simulink model "gm_interlock_deadtime_vnl"  (R2020b)
settings: Solver=FixedStepDiscrete  StartTime=0.0  StopTime=0.01  RelTol=1e-3
libraries: simulink x17, hdlmdlgenlib x12, hdlsllib x7, eePwmGeneratorTwoLevel x1, powerlib_meascontrol x1
(part 1 of 2)
settings Model: Creator=ts  LastModifiedBy=ts
settings DataIOCC: LimitDataPoints=on  SaveOutput=off  SaveTime=off
settings OptimizationCC: BlockReduction=off  ConditionallyExecuteInputs=off  DefaultParameterBehavior=Inlined  LifeSpan=inf
settings DebuggingCC: AlgebraicLoopMsg=error  InheritedTsInSrcMsg=none  SingleTaskRateTransMsg=error  AllowSymbolicDim=off  StrictBusMsg=ErrorOnBusTreatedAsVector  SFUnexpectedBacktrackingDiag=warning  SFNoUnconditionalDefaultTransitionDiag=warning  SFExecutionAtInitializationDiag=none  ArithmeticOperatorsInVariantConditions=warning
settings HardwareCC: ProdBitPerPointer=32  ProdBitPerSizeT=32  ProdBitPerPtrDiffT=32  ProdLargestAtomicFloat=None  ProdIntDivRoundTo=Undefined  ProdEndianess=Unspecified  ProdWordSize=32  ProdHWDeviceType=ASIC/FPGA->ASIC/FPGA  ProdEqTarget=off
settings SFSimCC: SimUseLocalCustomCode=off  CustomCodeUndefinedFunction=UseInterfaceOnly
settings RTWCC: RTWUseLocalCustomCode=off
settings CodeAppCC: StateflowObjectComments=on
settings GRTTargetCC: TargetLangStandard=C89/C90 (ANSI)
settings ConfigComp: CovScope=ReferencedModels  CovMetricSettings=dw  CovSaveCumulativeToWorkspaceVar=on  CovSaveSingleToWorkspaceVar=on  CovExternalEMLEnable=off  CovSFcnEnable=off

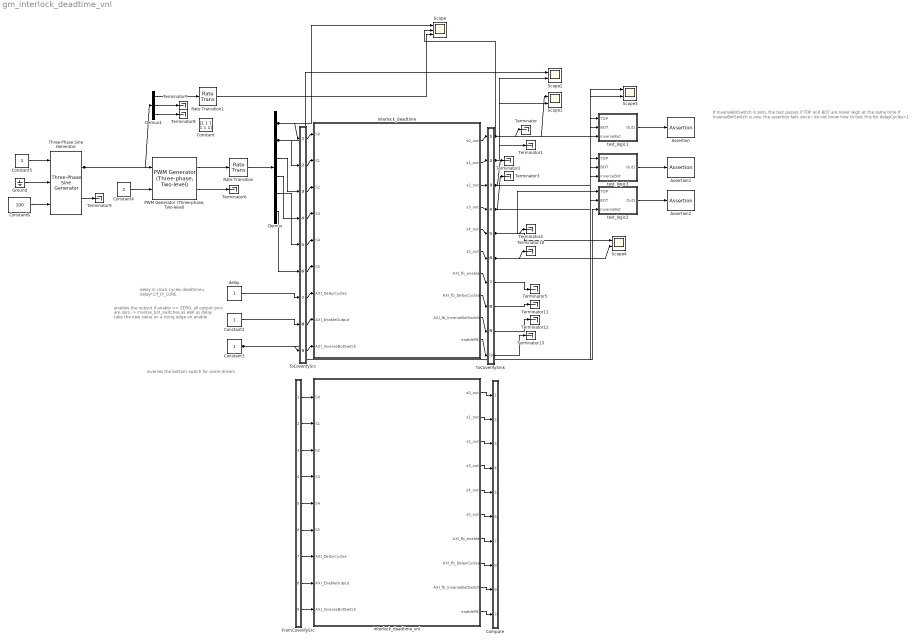
== system gm_interlock_deadtime_vnl ==
  note: If InverseBotSwitch is zero, the test passes if TOP and BOT are never High at the same time
      | If InverseBotSwitch is one, the assertion fails since I do not know how to test this for delayCycles>1
  note: enables the output
      | if enable == ZERO, all output pins are zero
      |
      | -> inverse_bot_switches as well as delay take the
      | new value on a rising edge on enable
  note: inverses the bottom switch for some drivers
  note: delay in clock cycles
      | deadtime= delay*1/f_IP_CORE
  Assertion : Assertion
  Assertion1 : Assertion
  Assertion2 : Assertion
  Compare : Subsystem
      mask Display: disp('')
  Constant : Constant  Value=[1 1 1 1 1 1]  OutDataTypeStr=boolean
  Constant2 : Constant  OutDataTypeStr=boolean  SampleTime=1/100e6
  Constant3 : Constant  OutDataTypeStr=boolean  SampleTime=1/100e6
  Constant4 : Constant  Value=2  SampleTime=-1
  Constant5 : Constant  SampleTime=-1
  Constant6 : Constant  Value=100  SampleTime=-1
  Demux : Demux  Outputs=6
  Demux1 : Demux  Outputs=3
  FromCoverifySrc : Subsystem
      mask Display: disp('')
  Ground : Ground
  "PWM Generator (Three-phase, Two-level)" : eePwmGeneratorTwoLevel/PWM Generator (Three-phase, Two-level)  PWMMode=Continuous PWM (CPWM)  CPWMMode=SPWM: sinusoidal PWM  DPWMMode=60 DPWM: 60 degree discontinuous PWM  fsw=10e3  Ts=1/(100*100e3)
      settings: SourceProductBaseCode=PS
  Rate Transition : RateTransition  OutPortSampleTime=1/100e6
  Rate Transition1 : RateTransition  OutPortSampleTime=1/100e6
  Scope : Scope  NumInputPorts=3
  Scope{1..4} (4 alike) : Scope  NumInputPorts=2
  Terminator{,1..13} (14 alike) : Terminator
  Three-Phase Sine Generator : powerlib_meascontrol/Pulse & Signal Generators/Three-Phase Sine Generator  Ts=1/100e3
      settings: SourceProductBaseCode=PS
  ToCoverifySink : Subsystem
      mask Display: disp('')
  ToCoverifySrc : Subsystem
      mask Display: disp('')
  delay : Constant  OutDataTypeStr=fixdt(0,10,0)  SampleTime=1/100e6
  interlock_deadtime : Subsystem  TreatAsAtomicUnit=on
  interlock_deadtime_vnl : Subsystem  TreatAsAtomicUnit=on
  test_logic1 : Subsystem
  test_logic2 : Subsystem
  test_logic3 : Subsystem
  wires:
  Constant4/1 -> "PWM Generator (Three-phase, Two-level)"/2
  Three-Phase Sine Generator/1 -> Demux1/1, "PWM Generator (Three-phase, Two-level)"/1
  Constant5/1 -> Three-Phase Sine Generator/1
  Constant6/1 -> Three-Phase Sine Generator/3
  Demux/1 -> Scope/1, ToCoverifySrc/1(in1)
  Demux/2 -> Scope2/1, ToCoverifySrc/2(in2)
  Demux1/1 -> Rate Transition1/1
  Rate Transition1/1 -> Scope/3
  Constant3/1 -> test_logic2/3(inverseBot), test_logic3/3(inverseBot), test_logic1/3(inverseBot), ToCoverifySrc/9(in9)
  "PWM Generator (Three-phase, Two-level)"/2 -> Terminator6/1
  Demux1/2 -> Terminator7/1
  Demux1/3 -> Terminator8/1
  Three-Phase Sine Generator/2 -> Terminator9/1
  Ground/1 -> Three-Phase Sine Generator/2
  test_logic3/1(Out1) -> Assertion1/1
  test_logic2/1(Out1) -> Assertion2/1
  test_logic1/1(Out1) -> Assertion/1
  Rate Transition/1 -> Demux/1
  "PWM Generator (Three-phase, Two-level)"/1 -> Rate Transition/1
  ToCoverifySrc/1(out1) -> interlock_deadtime/1(S0)
  ToCoverifySrc/2(out2) -> interlock_deadtime/2(S1)
  ToCoverifySrc/3(out3) -> interlock_deadtime/3(S2)
  ToCoverifySrc/4(out4) -> interlock_deadtime/4(S3)
  ToCoverifySrc/5(out5) -> interlock_deadtime/5(S4)
  ToCoverifySrc/6(out6) -> interlock_deadtime/6(S5)
  ToCoverifySrc/7(out7) -> interlock_deadtime/7(AXI_DelayCycles)
  ToCoverifySrc/8(out8) -> interlock_deadtime/8(AXI_EnableOutput)
  ToCoverifySrc/9(out9) -> interlock_deadtime/9(AXI_InverseBotSwitch)
  interlock_deadtime/1(s0_out) -> ToCoverifySink/1(in1)
  interlock_deadtime/2(s1_out) -> ToCoverifySink/2(in2)
  interlock_deadtime/3(s2_out) -> ToCoverifySink/3(in3)
  interlock_deadtime/4(s3_out) -> ToCoverifySink/4(in4)
  interlock_deadtime/5(s4_out) -> ToCoverifySink/5(in5)
  interlock_deadtime/6(s5_out) -> ToCoverifySink/6(in6)
  interlock_deadtime/7(AXI_fb_enable) -> ToCoverifySink/7(in7)
  interlock_deadtime/8(AXI_fb_DelayCycles) -> ToCoverifySink/8(in8)
  interlock_deadtime/9(AXI_fb_InverseBotSwitch) -> ToCoverifySink/9(in9)
  interlock_deadtime/10(enableFB) -> ToCoverifySink/10(in10)
  Demux/3 -> ToCoverifySrc/3(in3)
  Demux/4 -> ToCoverifySrc/4(in4)
  Demux/5 -> ToCoverifySrc/5(in5)
  Demux/6 -> ToCoverifySrc/6(in6)
  delay/1 -> ToCoverifySrc/7(in7)
  Constant2/1 -> ToCoverifySrc/8(in8)
  ToCoverifySink/1(out1) -> Scope1/1, Terminator/1, test_logic1/1(TOP), Scope/2
  ToCoverifySink/2(out2) -> Terminator1/1, test_logic1/2(BOT), Scope2/2, Scope1/2
  ToCoverifySink/3(out3) -> Terminator2/1, test_logic3/1(TOP), Scope3/1
  ToCoverifySink/4(out4) -> Terminator3/1, test_logic3/2(BOT), Scope3/2
  ToCoverifySink/5(out5) -> Terminator4/1, test_logic2/1(TOP), Scope4/1
  ToCoverifySink/6(out6) -> Terminator10/1, test_logic2/2(BOT), Scope4/2
  ToCoverifySink/7(out7) -> Terminator5/1
  ToCoverifySink/8(out8) -> Terminator11/1
  ToCoverifySink/9(out9) -> Terminator12/1
  ToCoverifySink/10(out10) -> Terminator13/1
  FromCoverifySrc/1(out1) -> interlock_deadtime_vnl/1(S0)
  FromCoverifySrc/2(out2) -> interlock_deadtime_vnl/2(S1)
  FromCoverifySrc/3(out3) -> interlock_deadtime_vnl/3(S2)
  FromCoverifySrc/4(out4) -> interlock_deadtime_vnl/4(S3)
  FromCoverifySrc/5(out5) -> interlock_deadtime_vnl/5(S4)
  FromCoverifySrc/6(out6) -> interlock_deadtime_vnl/6(S5)
  FromCoverifySrc/7(out7) -> interlock_deadtime_vnl/7(AXI_DelayCycles)
  FromCoverifySrc/8(out8) -> interlock_deadtime_vnl/8(AXI_EnableOutput)
  FromCoverifySrc/9(out9) -> interlock_deadtime_vnl/9(AXI_InverseBotSwitch)
  interlock_deadtime_vnl/1(s0_out) -> Compare/1(in1)
  interlock_deadtime_vnl/2(s1_out) -> Compare/2(in2)
  interlock_deadtime_vnl/3(s2_out) -> Compare/3(in3)
  interlock_deadtime_vnl/4(s3_out) -> Compare/4(in4)
  interlock_deadtime_vnl/5(s4_out) -> Compare/5(in5)
  interlock_deadtime_vnl/6(s5_out) -> Compare/6(in6)
  interlock_deadtime_vnl/7(AXI_fb_enable) -> Compare/7(in7)
  interlock_deadtime_vnl/8(AXI_fb_DelayCycles) -> Compare/8(in8)
  interlock_deadtime_vnl/9(AXI_fb_InverseBotSwitch) -> Compare/9(in9)
  interlock_deadtime_vnl/10(enableFB) -> Compare/10(in10)

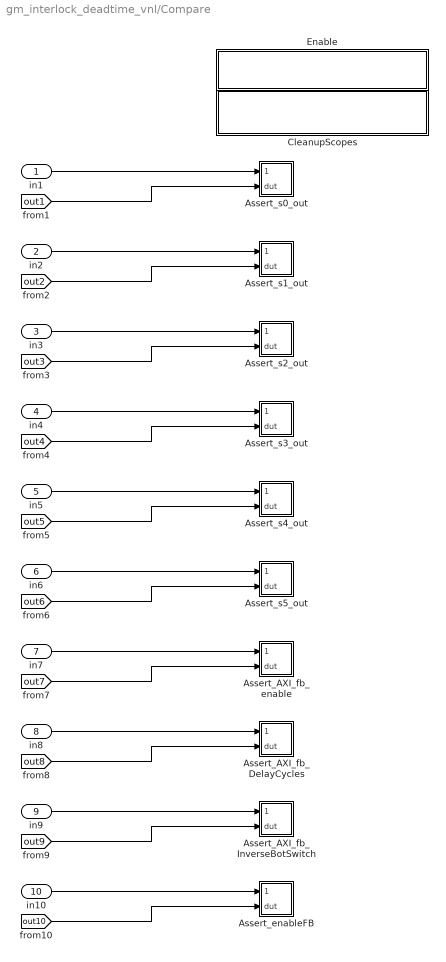
== system gm_interlock_deadtime_vnl/Compare ==
  in1 : Inport
  in2 : Inport  Port=2
  in3 : Inport  Port=3
  in4 : Inport  Port=4
  in5 : Inport  Port=5
  in6 : Inport  Port=6
  in7 : Inport  Port=7
  in8 : Inport  Port=8
  in9 : Inport  Port=9
  in10 : Inport  Port=10
  Assert_AXI_fb_DelayCycles : Subsystem
  Assert_AXI_fb_InverseBotSwitch : Subsystem
  Assert_AXI_fb_enable : Subsystem
  Assert_enableFB : Subsystem
  Assert_s0_out : Subsystem
  Assert_s1_out : Subsystem
  Assert_s2_out : Subsystem
  Assert_s3_out : Subsystem
  Assert_s4_out : Subsystem
  Assert_s5_out : Subsystem
  CleanupScopes : Subsystem
      settings: OpenFcn=|
      | blkName = gcb; %self block
      | idx = regexp(blkName, '/CleanupScopes$', 'once');
      | blkParent = blkName(1:idx-1);
      | blks=find_system(blkParent, 'LookUnderMasks', 'all','blocktype', 'Scope');
      | for itr = 1:length(blks)
      | 	 hScopeCfg = get_param(blks{itr},'ScopeConfiguration');
      | 	 hScopeCfg.Visible = ~ hScopeCfg.Visible;
      | end
      | drawnow;
      mask Display: fprintf(message('hdlcoder:cosim:vnl_dblclick').getString());
  Enable : Subsystem
      settings: OpenFcn=|
      | blkName = gcb;
      | idx = regexp(blkName, '/Enable$', 'once');
      | blkParent = blkName(1:idx-1);
      | blks=find_system(blkParent, 'LookUnderMasks', 'all','blocktype', 'Assertion');
      | e = get_param(blks{1}, 'Enabled');
      | if strcmp(e, 'on'), f= 'off';, else, f = 'on';, end
      | for ii=1:length(blks), set_param(blks{ii}, 'Enabled', f);, end
      | set_param(gcb, 'MaskDisplay',['fprintf(message(''hdlcoder:cosim:vnl_dblclick_assertions'',','''',upper(e),'''',').getString())']);
      mask Display: fprintf(message('hdlcoder:cosim:vnl_dblclick_assertions','OFF').getString());
  wires:
  in1/1 -> Assert_s0_out/1(cosim)
  [out1] -> Assert_s0_out/2(dut)
  in2/1 -> Assert_s1_out/1(cosim)
  [out2] -> Assert_s1_out/2(dut)
  in3/1 -> Assert_s2_out/1(cosim)
  [out3] -> Assert_s2_out/2(dut)
  in4/1 -> Assert_s3_out/1(cosim)
  [out4] -> Assert_s3_out/2(dut)
  in5/1 -> Assert_s4_out/1(cosim)
  [out5] -> Assert_s4_out/2(dut)
  in6/1 -> Assert_s5_out/1(cosim)
  [out6] -> Assert_s5_out/2(dut)
  in7/1 -> Assert_AXI_fb_enable/1(cosim)
  [out7] -> Assert_AXI_fb_enable/2(dut)
  in8/1 -> Assert_AXI_fb_DelayCycles/1(cosim)
  [out8] -> Assert_AXI_fb_DelayCycles/2(dut)
  in9/1 -> Assert_AXI_fb_InverseBotSwitch/1(cosim)
  [out9] -> Assert_AXI_fb_InverseBotSwitch/2(dut)
  in10/1 -> Assert_enableFB/1(cosim)
  [out10] -> Assert_enableFB/2(dut)

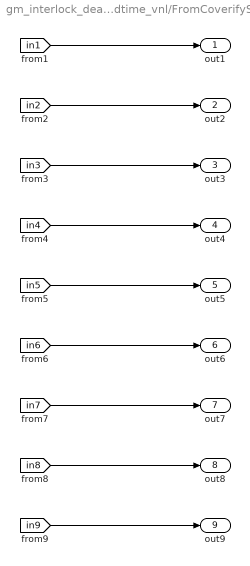
== system gm_interlock_deadtime_vnl/FromCoverifySrc ==
  out1 : Outport
  out2 : Outport  Port=2
  out3 : Outport  Port=3
  out4 : Outport  Port=4
  out5 : Outport  Port=5
  out6 : Outport  Port=6
  out7 : Outport  Port=7
  out8 : Outport  Port=8
  out9 : Outport  Port=9
  wires:
  [in1] -> out1/1
  [in2] -> out2/1
  [in3] -> out3/1
  [in4] -> out4/1
  [in5] -> out5/1
  [in6] -> out6/1
  [in7] -> out7/1
  [in8] -> out8/1
  [in9] -> out9/1

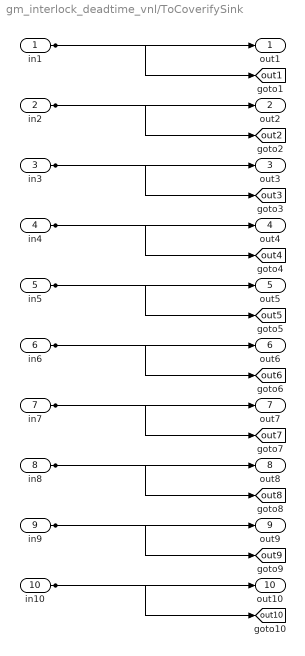
== system gm_interlock_deadtime_vnl/ToCoverifySink ==
  in1 : Inport
  in2 : Inport  Port=2
  in3 : Inport  Port=3
  in4 : Inport  Port=4
  in5 : Inport  Port=5
  in6 : Inport  Port=6
  in7 : Inport  Port=7
  in8 : Inport  Port=8
  in9 : Inport  Port=9
  in10 : Inport  Port=10
  out1 : Outport
  out2 : Outport  Port=2
  out3 : Outport  Port=3
  out4 : Outport  Port=4
  out5 : Outport  Port=5
  out6 : Outport  Port=6
  out7 : Outport  Port=7
  out8 : Outport  Port=8
  out9 : Outport  Port=9
  out10 : Outport  Port=10
  tag scope: out10=global, out1=global, out2=global, out3=global, out4=global, out5=global, out6=global, out7=global, out8=global, out9=global
  wires:
  in1/1 -> out1/1, [out1]
  in2/1 -> out2/1, [out2]
  in3/1 -> out3/1, [out3]
  in4/1 -> out4/1, [out4]
  in5/1 -> out5/1, [out5]
  in6/1 -> out6/1, [out6]
  in7/1 -> out7/1, [out7]
  in8/1 -> out8/1, [out8]
  in9/1 -> out9/1, [out9]
  in10/1 -> out10/1, [out10]

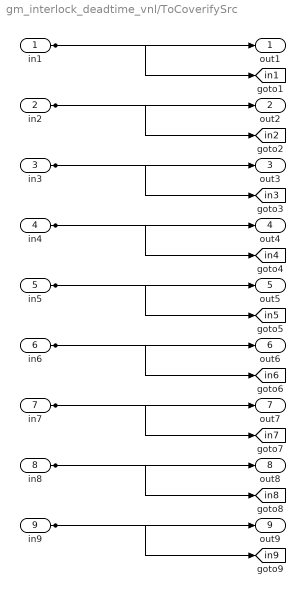
== system gm_interlock_deadtime_vnl/ToCoverifySrc ==
  in1 : Inport
  in2 : Inport  Port=2
  in3 : Inport  Port=3
  in4 : Inport  Port=4
  in5 : Inport  Port=5
  in6 : Inport  Port=6
  in7 : Inport  Port=7
  in8 : Inport  Port=8
  in9 : Inport  Port=9
  out1 : Outport
  out2 : Outport  Port=2
  out3 : Outport  Port=3
  out4 : Outport  Port=4
  out5 : Outport  Port=5
  out6 : Outport  Port=6
  out7 : Outport  Port=7
  out8 : Outport  Port=8
  out9 : Outport  Port=9
  tag scope: in1=global, in2=global, in3=global, in4=global, in5=global, in6=global, in7=global, in8=global, in9=global
  wires:
  in1/1 -> out1/1, [in1]
  in2/1 -> out2/1, [in2]
  in3/1 -> out3/1, [in3]
  in4/1 -> out4/1, [in4]
  in5/1 -> out5/1, [in5]
  in6/1 -> out6/1, [in6]
  in7/1 -> out7/1, [in7]
  in8/1 -> out8/1, [in8]
  in9/1 -> out9/1, [in9]

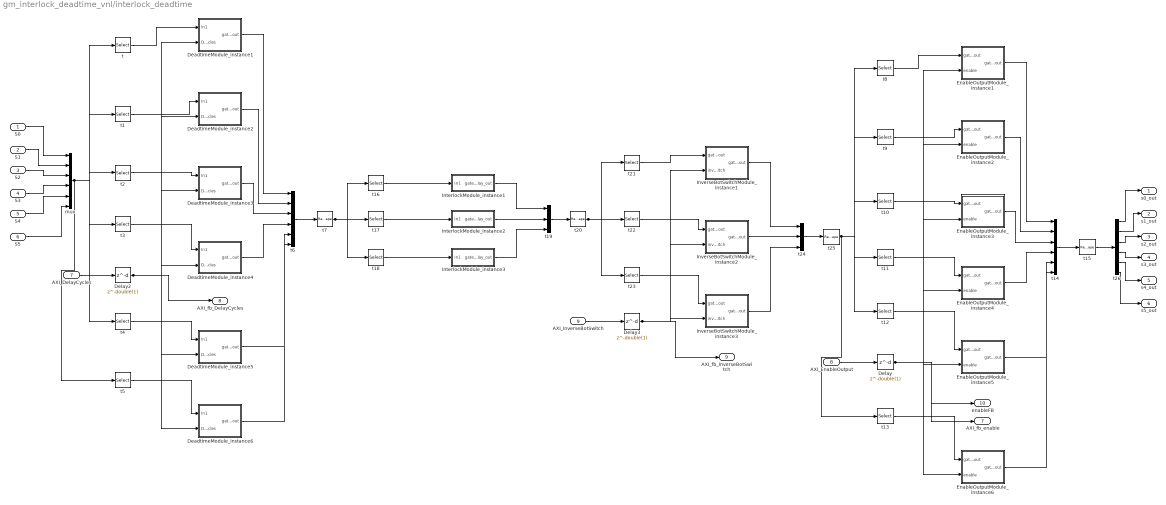
== system gm_interlock_deadtime_vnl/interlock_deadtime ==
  S0 : Inport  OutDataTypeStr=boolean  PortDimensions=1  SampleTime=1e-08
  S1 : Inport  Port=2  OutDataTypeStr=boolean  PortDimensions=1  SampleTime=1e-08
  S2 : Inport  Port=3  OutDataTypeStr=boolean  PortDimensions=1  SampleTime=1e-08
  S3 : Inport  Port=4  OutDataTypeStr=boolean  PortDimensions=1  SampleTime=1e-08
  S4 : Inport  Port=5  OutDataTypeStr=boolean  PortDimensions=1  SampleTime=1e-08
  S5 : Inport  Port=6  OutDataTypeStr=boolean  PortDimensions=1  SampleTime=1e-08
  AXI_DelayCycles : Inport  Port=7  OutDataTypeStr=fixdt(0, 10, 0)  PortDimensions=1  SampleTime=1e-08
  AXI_EnableOutput : Inport  Port=8  OutDataTypeStr=boolean  PortDimensions=1  SampleTime=1e-08
  AXI_InverseBotSwitch : Inport  Port=9  OutDataTypeStr=boolean  PortDimensions=1  SampleTime=1e-08
  DeadtimeModule_instance1 : Subsystem
  DeadtimeModule_instance2 : Subsystem
  DeadtimeModule_instance3 : Subsystem
  DeadtimeModule_instance4 : Subsystem
  DeadtimeModule_instance5 : Subsystem
  DeadtimeModule_instance6 : Subsystem
  Delay : Delay  DelayLength=double(1)  InitialCondition=0  SampleTime=1e-08
  Delay2 : Delay  DelayLength=double(1)  InitialCondition=0  SampleTime=1e-08
  Delay3 : Delay  DelayLength=double(1)  InitialCondition=0  SampleTime=1e-08
  EnableOutputModule_instance1 : Subsystem
  EnableOutputModule_instance2 : Subsystem
  EnableOutputModule_instance3 : Subsystem
  EnableOutputModule_instance4 : Subsystem
  EnableOutputModule_instance5 : Subsystem
  EnableOutputModule_instance6 : Subsystem
  InterlockModule_instance1 : Subsystem
  InterlockModule_instance2 : Subsystem
  InterlockModule_instance3 : Subsystem
  InverseBotSwitchModule_instance1 : Subsystem
  InverseBotSwitchModule_instance2 : Subsystem
  InverseBotSwitchModule_instance3 : Subsystem
  mux : Mux  Inputs=6
  t : Selector  SampleTime=1e-08  IndexOptions=Index vector (dialog)  Indices=double(1)  OutputSizes=1
  t1 : Selector  SampleTime=1e-08  IndexOptions=Index vector (dialog)  Indices=double(2)  OutputSizes=1
  t10 : Selector  SampleTime=1e-08  IndexOptions=Index vector (dialog)  Indices=double(3)  OutputSizes=1
  t11 : Selector  SampleTime=1e-08  IndexOptions=Index vector (dialog)  Indices=double(4)  OutputSizes=1
  t12 : Selector  SampleTime=1e-08  IndexOptions=Index vector (dialog)  Indices=double(5)  OutputSizes=1
  t13 : Selector  SampleTime=1e-08  IndexOptions=Index vector (dialog)  Indices=double(6)  OutputSizes=1
  t14 : Concatenate  NumInputs=6
  t{7,15,20,25} (4 alike) : Reshape
  t16 : Selector  SampleTime=1e-08  IndexOptions=Index vector (dialog)  Indices=double([1 2])  OutputSizes=1
  t17 : Selector  SampleTime=1e-08  IndexOptions=Index vector (dialog)  Indices=double([3 4])  OutputSizes=1
  t18 : Selector  SampleTime=1e-08  IndexOptions=Index vector (dialog)  Indices=double([5 6])  OutputSizes=1
  t19 : Concatenate  NumInputs=3
  t2 : Selector  SampleTime=1e-08  IndexOptions=Index vector (dialog)  Indices=double(3)  OutputSizes=1
  t21 : Selector  SampleTime=1e-08  IndexOptions=Index vector (dialog)  Indices=double([1 2])  OutputSizes=1
  t22 : Selector  SampleTime=1e-08  IndexOptions=Index vector (dialog)  Indices=double([3 4])  OutputSizes=1
  t23 : Selector  SampleTime=1e-08  IndexOptions=Index vector (dialog)  Indices=double([5 6])  OutputSizes=1
  t24 : Concatenate  NumInputs=3
  t26 : Demux  Outputs=6
  t3 : Selector  SampleTime=1e-08  IndexOptions=Index vector (dialog)  Indices=double(4)  OutputSizes=1
  t4 : Selector  SampleTime=1e-08  IndexOptions=Index vector (dialog)  Indices=double(5)  OutputSizes=1
  t5 : Selector  SampleTime=1e-08  IndexOptions=Index vector (dialog)  Indices=double(6)  OutputSizes=1
  t6 : Concatenate  NumInputs=6
  t8 : Selector  SampleTime=1e-08  IndexOptions=Index vector (dialog)  Indices=double(1)  OutputSizes=1
  t9 : Selector  SampleTime=1e-08  IndexOptions=Index vector (dialog)  Indices=double(2)  OutputSizes=1
  s0_out : Outport  VectorParamsAs1DForOutWhenUnconnected=off
  s1_out : Outport  Port=2  VectorParamsAs1DForOutWhenUnconnected=off
  s2_out : Outport  Port=3  VectorParamsAs1DForOutWhenUnconnected=off
  s3_out : Outport  Port=4  VectorParamsAs1DForOutWhenUnconnected=off
  s4_out : Outport  Port=5  VectorParamsAs1DForOutWhenUnconnected=off
  s5_out : Outport  Port=6  VectorParamsAs1DForOutWhenUnconnected=off
  AXI_fb_enable : Outport  Port=7  VectorParamsAs1DForOutWhenUnconnected=off
  AXI_fb_DelayCycles : Outport  Port=8  VectorParamsAs1DForOutWhenUnconnected=off
  AXI_fb_InverseBotSwitch : Outport  Port=9  VectorParamsAs1DForOutWhenUnconnected=off
  enableFB : Outport  Port=10  VectorParamsAs1DForOutWhenUnconnected=off
  wires:
  t26/6 -> s5_out/1
  t26/5 -> s4_out/1
  t26/4 -> s3_out/1
  t26/3 -> s2_out/1
  t26/2 -> s1_out/1
  t26/1 -> s0_out/1
  InverseBotSwitchModule_instance3/1(gate_enable_out) -> t24/3
  InverseBotSwitchModule_instance2/1(gate_enable_out) -> t24/2
  InverseBotSwitchModule_instance1/1(gate_enable_out) -> t24/1
  t24/1 -> t25/1
  t23/1 -> InverseBotSwitchModule_instance3/1(gate_delay_out)
  t22/1 -> InverseBotSwitchModule_instance2/1(gate_delay_out)
  t21/1 -> InverseBotSwitchModule_instance1/1(gate_delay_out)
  InterlockModule_instance3/1(gate_delay_out) -> t19/3
  InterlockModule_instance2/1(gate_delay_out) -> t19/2
  InterlockModule_instance1/1(gate_delay_out) -> t19/1
  t19/1 -> t20/1
  t18/1 -> InterlockModule_instance3/1(In1)
  t17/1 -> InterlockModule_instance2/1(In1)
  t16/1 -> InterlockModule_instance1/1(In1)
  EnableOutputModule_instance6/1(gate_enable_out) -> t14/6
  EnableOutputModule_instance5/1(gate_enable_out) -> t14/5
  EnableOutputModule_instance4/1(gate_enable_out) -> t14/4
  EnableOutputModule_instance3/1(gate_enable_out) -> t14/3
  EnableOutputModule_instance2/1(gate_enable_out) -> t14/2
  EnableOutputModule_instance1/1(gate_enable_out) -> t14/1
  t14/1 -> t15/1
  t13/1 -> EnableOutputModule_instance6/1(gate_delay_out)
  t12/1 -> EnableOutputModule_instance5/1(gate_delay_out)
  t11/1 -> EnableOutputModule_instance4/1(gate_delay_out)
  t10/1 -> EnableOutputModule_instance3/1(gate_delay_out)
  t9/1 -> EnableOutputModule_instance2/1(gate_delay_out)
  t8/1 -> EnableOutputModule_instance1/1(gate_delay_out)
  DeadtimeModule_instance6/1(gate_delay_out) -> t6/6
  DeadtimeModule_instance5/1(gate_delay_out) -> t6/5
  DeadtimeModule_instance4/1(gate_delay_out) -> t6/4
  DeadtimeModule_instance3/1(gate_delay_out) -> t6/3
  DeadtimeModule_instance2/1(gate_delay_out) -> t6/2
  DeadtimeModule_instance1/1(gate_delay_out) -> t6/1
  t6/1 -> t7/1
  t5/1 -> DeadtimeModule_instance6/1(In1)
  t4/1 -> DeadtimeModule_instance5/1(In1)
  t3/1 -> DeadtimeModule_instance4/1(In1)
  t2/1 -> DeadtimeModule_instance3/1(In1)
  t1/1 -> DeadtimeModule_instance2/1(In1)
  t/1 -> DeadtimeModule_instance1/1(In1)
  mux/1 -> t/1, t1/1, t2/1, t3/1, t4/1, t5/1
  t25/1 -> t8/1, t9/1, t10/1, t11/1, t12/1, t13/1
  t20/1 -> t21/1, t22/1, t23/1
  t15/1 -> t26/1
  Delay3/1 -> AXI_fb_InverseBotSwitch/1, InverseBotSwitchModule_instance1/2(inverse_bottom_switch), InverseBotSwitchModule_instance2/2(inverse_bottom_switch), InverseBotSwitchModule_instance3/2(inverse_bottom_switch)
  Delay2/1 -> AXI_fb_DelayCycles/1, DeadtimeModule_instance1/2(DelayCycles), DeadtimeModule_instance2/2(DelayCycles), DeadtimeModule_instance3/2(DelayCycles), DeadtimeModule_instance4/2(DelayCycles), DeadtimeModule_instance5/2(DelayCycles), DeadtimeModule_instance6/2(DelayCycles)
  Delay/1 -> enableFB/1, AXI_fb_enable/1, EnableOutputModule_instance1/2(enable), EnableOutputModule_instance2/2(enable), EnableOutputModule_instance3/2(enable), EnableOutputModule_instance4/2(enable), EnableOutputModule_instance5/2(enable), EnableOutputModule_instance6/2(enable)
  t7/1 -> t16/1, t17/1, t18/1
  AXI_InverseBotSwitch/1 -> Delay3/1
  AXI_EnableOutput/1 -> Delay/1
  AXI_DelayCycles/1 -> Delay2/1
  S5/1 -> mux/6
  S4/1 -> mux/5
  S3/1 -> mux/4
  S2/1 -> mux/3
  S1/1 -> mux/2
  S0/1 -> mux/1

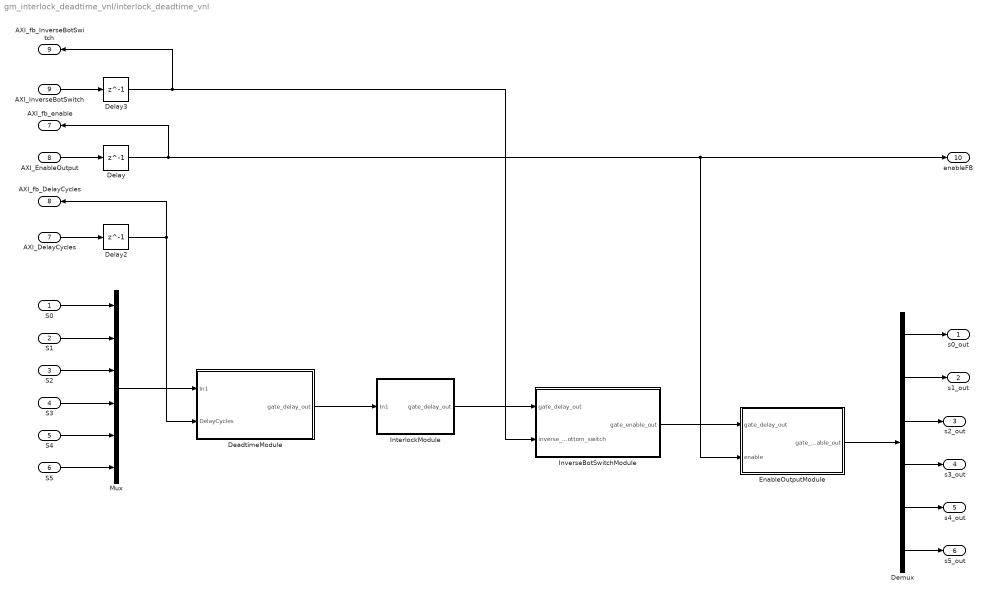
== system gm_interlock_deadtime_vnl/interlock_deadtime_vnl ==
  S0 : Inport
  S1 : Inport  Port=2
  S2 : Inport  Port=3
  S3 : Inport  Port=4
  S4 : Inport  Port=5
  S5 : Inport  Port=6
  AXI_DelayCycles : Inport  Port=7
  AXI_EnableOutput : Inport  Port=8
  AXI_InverseBotSwitch : Inport  Port=9
  DeadtimeModule : Subsystem  TreatAsAtomicUnit=on
  Delay : Delay  DelayLength=1
  Delay2 : Delay  DelayLength=1
  Delay3 : Delay  DelayLength=1
  Demux : Demux  Outputs=6
  EnableOutputModule : Subsystem  TreatAsAtomicUnit=on
  InterlockModule : Subsystem  TreatAsAtomicUnit=on
  InverseBotSwitchModule : Subsystem  TreatAsAtomicUnit=on
  Mux : Mux  Inputs=6
  s0_out : Outport  VectorParamsAs1DForOutWhenUnconnected=off
  s1_out : Outport  Port=2  VectorParamsAs1DForOutWhenUnconnected=off
  s2_out : Outport  Port=3  VectorParamsAs1DForOutWhenUnconnected=off
  s3_out : Outport  Port=4  VectorParamsAs1DForOutWhenUnconnected=off
  s4_out : Outport  Port=5  VectorParamsAs1DForOutWhenUnconnected=off
  s5_out : Outport  Port=6  VectorParamsAs1DForOutWhenUnconnected=off
  AXI_fb_enable : Outport  Port=7  VectorParamsAs1DForOutWhenUnconnected=off
  AXI_fb_DelayCycles : Outport  Port=8  VectorParamsAs1DForOutWhenUnconnected=off
  AXI_fb_InverseBotSwitch : Outport  Port=9  VectorParamsAs1DForOutWhenUnconnected=off
  enableFB : Outport  Port=10  VectorParamsAs1DForOutWhenUnconnected=off
  wires:
  AXI_DelayCycles/1 -> Delay2/1
  InverseBotSwitchModule/1(gate_enable_out) -> EnableOutputModule/1(gate_delay_out)
  InterlockModule/1(gate_delay_out) -> InverseBotSwitchModule/1(gate_delay_out)
  Delay/1 -> EnableOutputModule/2(enable), enableFB/1, AXI_fb_enable/1
  EnableOutputModule/1(gate_enable_out) -> Demux/1
  Demux/6 -> s5_out/1
  Demux/5 -> s4_out/1
  Demux/4 -> s3_out/1
  Demux/3 -> s2_out/1
  Demux/1 -> s0_out/1
  Demux/2 -> s1_out/1
  S5/1 -> Mux/6
  S4/1 -> Mux/5
  S3/1 -> Mux/4
  S2/1 -> Mux/3
  S1/1 -> Mux/2
  S0/1 -> Mux/1
  DeadtimeModule/1(gate_delay_out) -> InterlockModule/1(In1)
  Mux/1 -> DeadtimeModule/1(In1)
  Delay2/1 -> DeadtimeModule/2(DelayCycles), AXI_fb_DelayCycles/1
  AXI_EnableOutput/1 -> Delay/1
  Delay3/1 -> AXI_fb_InverseBotSwitch/1, InverseBotSwitchModule/2(inverse_bottom_switch)
  AXI_InverseBotSwitch/1 -> Delay3/1

== system gm_interlock_deadtime_vnl/test_logic1 ==
  TOP : Inport
  BOT : Inport  Port=2
  inverseBot : Inport  Port=3
  AND : Logic  IconShape=distinctive  AllPortsSameDT=off  OutDataTypeStr=boolean
  Constant : Constant
  NOT : Logic  Operator=NOT  IconShape=distinctive  AllPortsSameDT=off  OutDataTypeStr=boolean
  Switch : Switch  Criteria=u2 ~= 0
  Out1 : Outport
  wires:
  Constant/1 -> Switch/1
  Switch/1 -> Out1/1
  AND/1 -> NOT/1
  inverseBot/1 -> Switch/2
  NOT/1 -> Switch/3
  TOP/1 -> AND/1
  BOT/1 -> AND/2

== system gm_interlock_deadtime_vnl/test_logic2 ==
  TOP : Inport
  BOT : Inport  Port=2
  inverseBot : Inport  Port=3
  AND : Logic  IconShape=distinctive  AllPortsSameDT=off  OutDataTypeStr=boolean
  Constant : Constant
  NOT : Logic  Operator=NOT  IconShape=distinctive  AllPortsSameDT=off  OutDataTypeStr=boolean
  Switch : Switch  Criteria=u2 ~= 0
  Out1 : Outport
  wires:
  BOT/1 -> AND/2
  TOP/1 -> AND/1
  NOT/1 -> Switch/3
  inverseBot/1 -> Switch/2
  AND/1 -> NOT/1
  Switch/1 -> Out1/1
  Constant/1 -> Switch/1

== system gm_interlock_deadtime_vnl/test_logic3 ==
  TOP : Inport
  BOT : Inport  Port=2
  inverseBot : Inport  Port=3
  AND : Logic  IconShape=distinctive  AllPortsSameDT=off  OutDataTypeStr=boolean
  Constant : Constant
  NOT : Logic  Operator=NOT  IconShape=distinctive  AllPortsSameDT=off  OutDataTypeStr=boolean
  Switch : Switch  Criteria=u2 ~= 0
  Out1 : Outport
  wires:
  Constant/1 -> Switch/1
  Switch/1 -> Out1/1
  AND/1 -> NOT/1
  inverseBot/1 -> Switch/2
  NOT/1 -> Switch/3
  TOP/1 -> AND/1
  BOT/1 -> AND/2

== system gm_interlock_deadtime_vnl/Compare/Assert_AXI_fb_DelayCycles ==
  cosim : Inport
  dut : Inport  Port=2
  AssertEq : Assertion  StopWhenAssertionFail=off
  Compare To Zero : simulink/Logic and Bit Operations/Compare To Zero  relop===  OutDataTypeStr=boolean
  Relational Operator : RelationalOperator  Operator===  OutDataTypeStr=boolean  RndMeth=Nearest
  compare: AXI_fb_DelayCycles : Scope  NumInputPorts=3
  wires:
  Compare To Zero/1 -> compare: AXI_fb_DelayCycles/3  "err"
  Relational Operator/1 -> Compare To Zero/1, AssertEq/1
  cosim/1 -> compare: AXI_fb_DelayCycles/1, Relational Operator/1  "cosim"
  dut/1 -> compare: AXI_fb_DelayCycles/2, Relational Operator/2  "dut ref"

== system gm_interlock_deadtime_vnl/Compare/Assert_AXI_fb_InverseBotSwitch ==
  cosim : Inport
  dut : Inport  Port=2
  AssertEq : Assertion  StopWhenAssertionFail=off
  Compare To Zero : simulink/Logic and Bit Operations/Compare To Zero  relop===  OutDataTypeStr=boolean
  Relational Operator : RelationalOperator  Operator===  OutDataTypeStr=boolean  RndMeth=Nearest
  compare: AXI_fb_InverseBotSwitch : Scope  NumInputPorts=3
  wires:
  Compare To Zero/1 -> compare: AXI_fb_InverseBotSwitch/3  "err"
  Relational Operator/1 -> Compare To Zero/1, AssertEq/1
  cosim/1 -> compare: AXI_fb_InverseBotSwitch/1, Relational Operator/1  "cosim"
  dut/1 -> compare: AXI_fb_InverseBotSwitch/2, Relational Operator/2  "dut ref"

== system gm_interlock_deadtime_vnl/Compare/Assert_AXI_fb_enable ==
  cosim : Inport
  dut : Inport  Port=2
  AssertEq : Assertion  StopWhenAssertionFail=off
  Compare To Zero : simulink/Logic and Bit Operations/Compare To Zero  relop===  OutDataTypeStr=boolean
  Relational Operator : RelationalOperator  Operator===  OutDataTypeStr=boolean  RndMeth=Nearest
  compare: AXI_fb_enable : Scope  NumInputPorts=3
  wires:
  Compare To Zero/1 -> compare: AXI_fb_enable/3  "err"
  Relational Operator/1 -> Compare To Zero/1, AssertEq/1
  cosim/1 -> compare: AXI_fb_enable/1, Relational Operator/1  "cosim"
  dut/1 -> compare: AXI_fb_enable/2, Relational Operator/2  "dut ref"

== system gm_interlock_deadtime_vnl/Compare/Assert_enableFB ==
  cosim : Inport
  dut : Inport  Port=2
  AssertEq : Assertion  StopWhenAssertionFail=off
  Compare To Zero : simulink/Logic and Bit Operations/Compare To Zero  relop===  OutDataTypeStr=boolean
  Relational Operator : RelationalOperator  Operator===  OutDataTypeStr=boolean  RndMeth=Nearest
  compare: enableFB : Scope  NumInputPorts=3
  wires:
  Compare To Zero/1 -> compare: enableFB/3  "err"
  Relational Operator/1 -> Compare To Zero/1, AssertEq/1
  cosim/1 -> compare: enableFB/1, Relational Operator/1  "cosim"
  dut/1 -> compare: enableFB/2, Relational Operator/2  "dut ref"

== system gm_interlock_deadtime_vnl/Compare/Assert_s0_out ==
  cosim : Inport
  dut : Inport  Port=2
  AssertEq : Assertion  StopWhenAssertionFail=off
  Compare To Zero : simulink/Logic and Bit Operations/Compare To Zero  relop===  OutDataTypeStr=boolean
  Relational Operator : RelationalOperator  Operator===  OutDataTypeStr=boolean  RndMeth=Nearest
  compare: s0_out : Scope  NumInputPorts=3
  wires:
  Compare To Zero/1 -> compare: s0_out/3  "err"
  Relational Operator/1 -> Compare To Zero/1, AssertEq/1
  cosim/1 -> compare: s0_out/1, Relational Operator/1  "cosim"
  dut/1 -> compare: s0_out/2, Relational Operator/2  "dut ref"

== system gm_interlock_deadtime_vnl/Compare/Assert_s1_out ==
  cosim : Inport
  dut : Inport  Port=2
  AssertEq : Assertion  StopWhenAssertionFail=off
  Compare To Zero : simulink/Logic and Bit Operations/Compare To Zero  relop===  OutDataTypeStr=boolean
  Relational Operator : RelationalOperator  Operator===  OutDataTypeStr=boolean  RndMeth=Nearest
  compare: s1_out : Scope  NumInputPorts=3
  wires:
  Compare To Zero/1 -> compare: s1_out/3  "err"
  Relational Operator/1 -> Compare To Zero/1, AssertEq/1
  cosim/1 -> compare: s1_out/1, Relational Operator/1  "cosim"
  dut/1 -> compare: s1_out/2, Relational Operator/2  "dut ref"

== system gm_interlock_deadtime_vnl/Compare/Assert_s2_out ==
  cosim : Inport
  dut : Inport  Port=2
  AssertEq : Assertion  StopWhenAssertionFail=off
  Compare To Zero : simulink/Logic and Bit Operations/Compare To Zero  relop===  OutDataTypeStr=boolean
  Relational Operator : RelationalOperator  Operator===  OutDataTypeStr=boolean  RndMeth=Nearest
  compare: s2_out : Scope  NumInputPorts=3
  wires:
  Compare To Zero/1 -> compare: s2_out/3  "err"
  Relational Operator/1 -> Compare To Zero/1, AssertEq/1
  cosim/1 -> compare: s2_out/1, Relational Operator/1  "cosim"
  dut/1 -> compare: s2_out/2, Relational Operator/2  "dut ref"

== system gm_interlock_deadtime_vnl/Compare/Assert_s3_out ==
  cosim : Inport
  dut : Inport  Port=2
  AssertEq : Assertion  StopWhenAssertionFail=off
  Compare To Zero : simulink/Logic and Bit Operations/Compare To Zero  relop===  OutDataTypeStr=boolean
  Relational Operator : RelationalOperator  Operator===  OutDataTypeStr=boolean  RndMeth=Nearest
  compare: s3_out : Scope  NumInputPorts=3
  wires:
  Compare To Zero/1 -> compare: s3_out/3  "err"
  Relational Operator/1 -> Compare To Zero/1, AssertEq/1
  cosim/1 -> compare: s3_out/1, Relational Operator/1  "cosim"
  dut/1 -> compare: s3_out/2, Relational Operator/2  "dut ref"

== system gm_interlock_deadtime_vnl/Compare/Assert_s4_out ==
  cosim : Inport
  dut : Inport  Port=2
  AssertEq : Assertion  StopWhenAssertionFail=off
  Compare To Zero : simulink/Logic and Bit Operations/Compare To Zero  relop===  OutDataTypeStr=boolean
  Relational Operator : RelationalOperator  Operator===  OutDataTypeStr=boolean  RndMeth=Nearest
  compare: s4_out : Scope  NumInputPorts=3
  wires:
  Compare To Zero/1 -> compare: s4_out/3  "err"
  Relational Operator/1 -> Compare To Zero/1, AssertEq/1
  cosim/1 -> compare: s4_out/1, Relational Operator/1  "cosim"
  dut/1 -> compare: s4_out/2, Relational Operator/2  "dut ref"

== system gm_interlock_deadtime_vnl/Compare/Assert_s5_out ==
  cosim : Inport
  dut : Inport  Port=2
  AssertEq : Assertion  StopWhenAssertionFail=off
  Compare To Zero : simulink/Logic and Bit Operations/Compare To Zero  relop===  OutDataTypeStr=boolean
  Relational Operator : RelationalOperator  Operator===  OutDataTypeStr=boolean  RndMeth=Nearest
  compare: s5_out : Scope  NumInputPorts=3
  wires:
  Compare To Zero/1 -> compare: s5_out/3  "err"
  Relational Operator/1 -> Compare To Zero/1, AssertEq/1
  cosim/1 -> compare: s5_out/1, Relational Operator/1  "cosim"
  dut/1 -> compare: s5_out/2, Relational Operator/2  "dut ref"

== system gm_interlock_deadtime_vnl/Compare/CleanupScopes ==

== system gm_interlock_deadtime_vnl/Compare/Enable ==

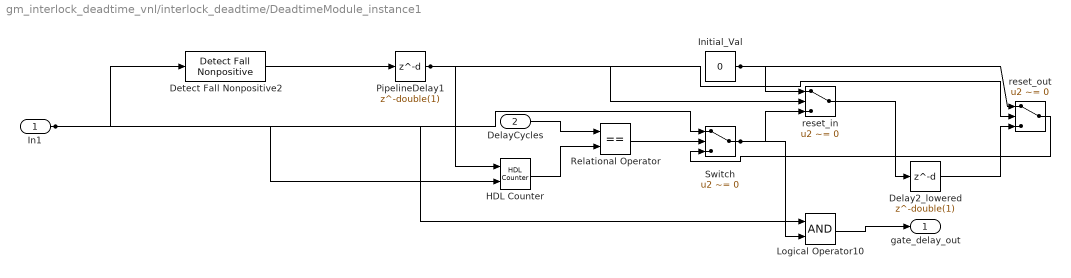
== system gm_interlock_deadtime_vnl/interlock_deadtime/DeadtimeModule_instance1 ==
  In1 : Inport  OutDataTypeStr=boolean  PortDimensions=1  SampleTime=1e-08
  DelayCycles : Inport  Port=2  OutDataTypeStr=fixdt(0, 10, 0)  PortDimensions=1  SampleTime=1e-08
  Delay2_lowered : Delay  DelayLength=double(1)  InitialCondition=0  SampleTime=1e-08
  Detect Fall Nonpositive2 : simulink/Logic and Bit Operations/Detect Fall Nonpositive  vinit=0  OutDataTypeStr=boolean
      settings: SourceProductBaseCode=SL
  HDL Counter : hdlsllib/Sources/HDL Counter  CountType=Free running  CountInit=double(0)  CountStep=double(1)  CountMax=25  CountFromType=Initial value  CountFrom=double(0)  CountResetPort=on  CountLoadPort=off  CountEnbPort=on  CountDirPort=off  CountDataType=Unsigned  CountWordLen=10  CountFracLen=0  CountSampTime=1e-08
  Initial_Val : Constant  Value=0  OutDataTypeStr=boolean  SampleTime=1e-08
  Logical Operator10 : Logic  AllPortsSameDT=off  OutDataTypeStr=boolean  SampleTime=1e-08
  PipelineDelay1 : Delay  DelayLength=double(1)  InitialCondition=0  SampleTime=1e-08
  Relational Operator : RelationalOperator  Operator===  OutDataTypeStr=boolean  SampleTime=1e-08  RndMeth=Nearest
  Switch : Switch  Criteria=u2 ~= 0  Threshold=double(0)  OutDataTypeStr=boolean  SampleTime=1e-08
  reset_in : Switch  Criteria=u2 ~= 0  Threshold=double(0)  OutDataTypeStr=boolean  SampleTime=1e-08
  reset_out : Switch  Criteria=u2 ~= 0  Threshold=double(0)  OutDataTypeStr=boolean  SampleTime=1e-08
  gate_delay_out : Outport
  wires:
  reset_in/1 -> Delay2_lowered/1
  Delay2_lowered/1 -> reset_out/3
  Initial_Val/1 -> reset_in/1, reset_out/1
  reset_out/1 -> Switch/3
  Detect Fall Nonpositive2/1 -> PipelineDelay1/1
  HDL Counter/1 -> Relational Operator/2
  Logical Operator10/1 -> gate_delay_out/1
  PipelineDelay1/1 -> HDL Counter/1, reset_in/2, reset_out/2
  Relational Operator/1 -> Switch/2
  Switch/1 -> reset_in/3, Logical Operator10/2
  DelayCycles/1 -> Relational Operator/1
  In1/1 -> Detect Fall Nonpositive2/1, HDL Counter/2, Switch/1, Logical Operator10/1

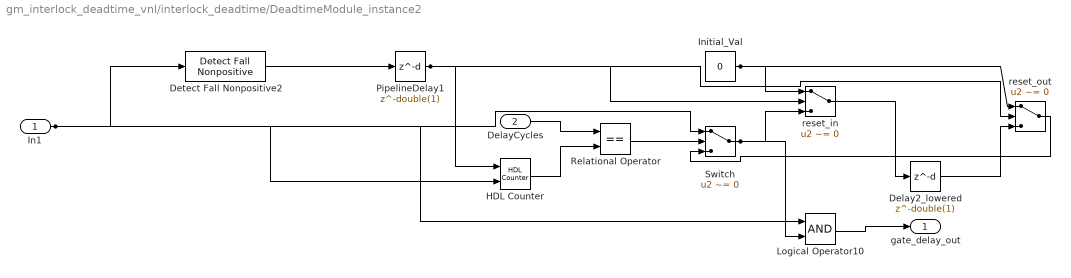
== system gm_interlock_deadtime_vnl/interlock_deadtime/DeadtimeModule_instance2 ==
  In1 : Inport  OutDataTypeStr=boolean  PortDimensions=1  SampleTime=1e-08
  DelayCycles : Inport  Port=2  OutDataTypeStr=fixdt(0, 10, 0)  PortDimensions=1  SampleTime=1e-08
  Delay2_lowered : Delay  DelayLength=double(1)  InitialCondition=0  SampleTime=1e-08
  Detect Fall Nonpositive2 : simulink/Logic and Bit Operations/Detect Fall Nonpositive  vinit=0  OutDataTypeStr=boolean
      settings: SourceProductBaseCode=SL
  HDL Counter : hdlsllib/Sources/HDL Counter  CountType=Free running  CountInit=double(0)  CountStep=double(1)  CountMax=25  CountFromType=Initial value  CountFrom=double(0)  CountResetPort=on  CountLoadPort=off  CountEnbPort=on  CountDirPort=off  CountDataType=Unsigned  CountWordLen=10  CountFracLen=0  CountSampTime=1e-08
  Initial_Val : Constant  Value=0  OutDataTypeStr=boolean  SampleTime=1e-08
  Logical Operator10 : Logic  AllPortsSameDT=off  OutDataTypeStr=boolean  SampleTime=1e-08
  PipelineDelay1 : Delay  DelayLength=double(1)  InitialCondition=0  SampleTime=1e-08
  Relational Operator : RelationalOperator  Operator===  OutDataTypeStr=boolean  SampleTime=1e-08  RndMeth=Nearest
  Switch : Switch  Criteria=u2 ~= 0  Threshold=double(0)  OutDataTypeStr=boolean  SampleTime=1e-08
  reset_in : Switch  Criteria=u2 ~= 0  Threshold=double(0)  OutDataTypeStr=boolean  SampleTime=1e-08
  reset_out : Switch  Criteria=u2 ~= 0  Threshold=double(0)  OutDataTypeStr=boolean  SampleTime=1e-08
  gate_delay_out : Outport
  wires:
  In1/1 -> Logical Operator10/1, Switch/1, HDL Counter/2, Detect Fall Nonpositive2/1
  DelayCycles/1 -> Relational Operator/1
  Switch/1 -> Logical Operator10/2, reset_in/3
  Relational Operator/1 -> Switch/2
  PipelineDelay1/1 -> reset_out/2, reset_in/2, HDL Counter/1
  Logical Operator10/1 -> gate_delay_out/1
  HDL Counter/1 -> Relational Operator/2
  Detect Fall Nonpositive2/1 -> PipelineDelay1/1
  reset_out/1 -> Switch/3
  Initial_Val/1 -> reset_out/1, reset_in/1
  Delay2_lowered/1 -> reset_out/3
  reset_in/1 -> Delay2_lowered/1

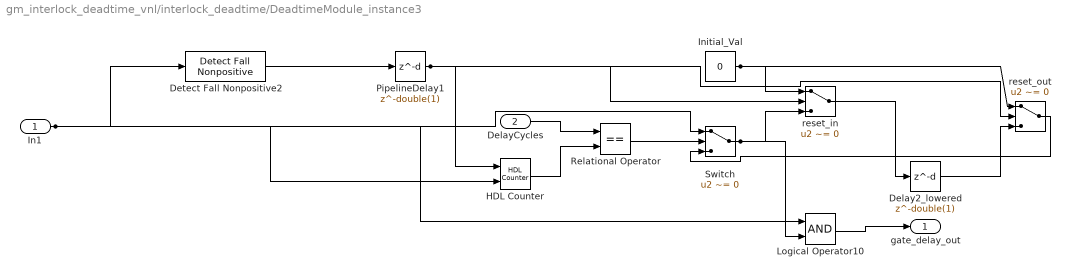
== system gm_interlock_deadtime_vnl/interlock_deadtime/DeadtimeModule_instance3 ==
  In1 : Inport  OutDataTypeStr=boolean  PortDimensions=1  SampleTime=1e-08
  DelayCycles : Inport  Port=2  OutDataTypeStr=fixdt(0, 10, 0)  PortDimensions=1  SampleTime=1e-08
  Delay2_lowered : Delay  DelayLength=double(1)  InitialCondition=0  SampleTime=1e-08
  Detect Fall Nonpositive2 : simulink/Logic and Bit Operations/Detect Fall Nonpositive  vinit=0  OutDataTypeStr=boolean
      settings: SourceProductBaseCode=SL
  HDL Counter : hdlsllib/Sources/HDL Counter  CountType=Free running  CountInit=double(0)  CountStep=double(1)  CountMax=25  CountFromType=Initial value  CountFrom=double(0)  CountResetPort=on  CountLoadPort=off  CountEnbPort=on  CountDirPort=off  CountDataType=Unsigned  CountWordLen=10  CountFracLen=0  CountSampTime=1e-08
  Initial_Val : Constant  Value=0  OutDataTypeStr=boolean  SampleTime=1e-08
  Logical Operator10 : Logic  AllPortsSameDT=off  OutDataTypeStr=boolean  SampleTime=1e-08
  PipelineDelay1 : Delay  DelayLength=double(1)  InitialCondition=0  SampleTime=1e-08
  Relational Operator : RelationalOperator  Operator===  OutDataTypeStr=boolean  SampleTime=1e-08  RndMeth=Nearest
  Switch : Switch  Criteria=u2 ~= 0  Threshold=double(0)  OutDataTypeStr=boolean  SampleTime=1e-08
  reset_in : Switch  Criteria=u2 ~= 0  Threshold=double(0)  OutDataTypeStr=boolean  SampleTime=1e-08
  reset_out : Switch  Criteria=u2 ~= 0  Threshold=double(0)  OutDataTypeStr=boolean  SampleTime=1e-08
  gate_delay_out : Outport
  wires:
  In1/1 -> Logical Operator10/1, Switch/1, HDL Counter/2, Detect Fall Nonpositive2/1
  DelayCycles/1 -> Relational Operator/1
  Switch/1 -> Logical Operator10/2, reset_in/3
  Relational Operator/1 -> Switch/2
  PipelineDelay1/1 -> reset_out/2, reset_in/2, HDL Counter/1
  Logical Operator10/1 -> gate_delay_out/1
  HDL Counter/1 -> Relational Operator/2
  Detect Fall Nonpositive2/1 -> PipelineDelay1/1
  reset_out/1 -> Switch/3
  Initial_Val/1 -> reset_out/1, reset_in/1
  Delay2_lowered/1 -> reset_out/3
  reset_in/1 -> Delay2_lowered/1

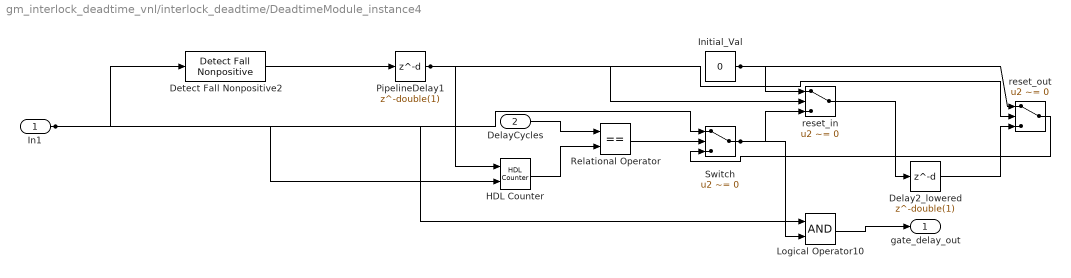
== system gm_interlock_deadtime_vnl/interlock_deadtime/DeadtimeModule_instance4 ==
  In1 : Inport  OutDataTypeStr=boolean  PortDimensions=1  SampleTime=1e-08
  DelayCycles : Inport  Port=2  OutDataTypeStr=fixdt(0, 10, 0)  PortDimensions=1  SampleTime=1e-08
  Delay2_lowered : Delay  DelayLength=double(1)  InitialCondition=0  SampleTime=1e-08
  Detect Fall Nonpositive2 : simulink/Logic and Bit Operations/Detect Fall Nonpositive  vinit=0  OutDataTypeStr=boolean
      settings: SourceProductBaseCode=SL
  HDL Counter : hdlsllib/Sources/HDL Counter  CountType=Free running  CountInit=double(0)  CountStep=double(1)  CountMax=25  CountFromType=Initial value  CountFrom=double(0)  CountResetPort=on  CountLoadPort=off  CountEnbPort=on  CountDirPort=off  CountDataType=Unsigned  CountWordLen=10  CountFracLen=0  CountSampTime=1e-08
  Initial_Val : Constant  Value=0  OutDataTypeStr=boolean  SampleTime=1e-08
  Logical Operator10 : Logic  AllPortsSameDT=off  OutDataTypeStr=boolean  SampleTime=1e-08
  PipelineDelay1 : Delay  DelayLength=double(1)  InitialCondition=0  SampleTime=1e-08
  Relational Operator : RelationalOperator  Operator===  OutDataTypeStr=boolean  SampleTime=1e-08  RndMeth=Nearest
  Switch : Switch  Criteria=u2 ~= 0  Threshold=double(0)  OutDataTypeStr=boolean  SampleTime=1e-08
  reset_in : Switch  Criteria=u2 ~= 0  Threshold=double(0)  OutDataTypeStr=boolean  SampleTime=1e-08
  reset_out : Switch  Criteria=u2 ~= 0  Threshold=double(0)  OutDataTypeStr=boolean  SampleTime=1e-08
  gate_delay_out : Outport
  wires:
  In1/1 -> Logical Operator10/1, Switch/1, HDL Counter/2, Detect Fall Nonpositive2/1
  DelayCycles/1 -> Relational Operator/1
  Switch/1 -> Logical Operator10/2, reset_in/3
  Relational Operator/1 -> Switch/2
  PipelineDelay1/1 -> reset_out/2, reset_in/2, HDL Counter/1
  Logical Operator10/1 -> gate_delay_out/1
  HDL Counter/1 -> Relational Operator/2
  Detect Fall Nonpositive2/1 -> PipelineDelay1/1
  reset_out/1 -> Switch/3
  Initial_Val/1 -> reset_out/1, reset_in/1
  Delay2_lowered/1 -> reset_out/3
  reset_in/1 -> Delay2_lowered/1

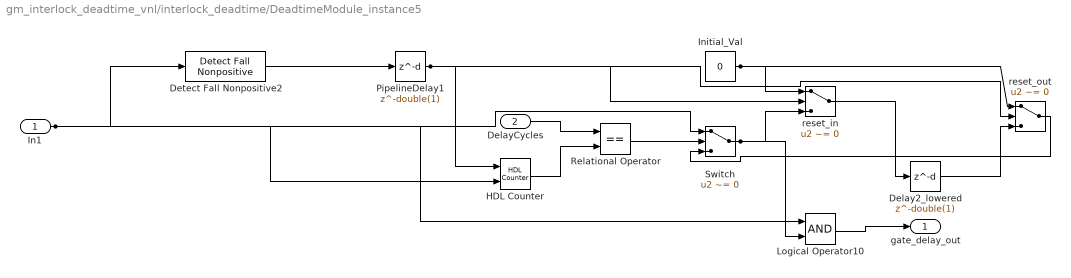
== system gm_interlock_deadtime_vnl/interlock_deadtime/DeadtimeModule_instance5 ==
  In1 : Inport  OutDataTypeStr=boolean  PortDimensions=1  SampleTime=1e-08
  DelayCycles : Inport  Port=2  OutDataTypeStr=fixdt(0, 10, 0)  PortDimensions=1  SampleTime=1e-08
  Delay2_lowered : Delay  DelayLength=double(1)  InitialCondition=0  SampleTime=1e-08
  Detect Fall Nonpositive2 : simulink/Logic and Bit Operations/Detect Fall Nonpositive  vinit=0  OutDataTypeStr=boolean
      settings: SourceProductBaseCode=SL
  HDL Counter : hdlsllib/Sources/HDL Counter  CountType=Free running  CountInit=double(0)  CountStep=double(1)  CountMax=25  CountFromType=Initial value  CountFrom=double(0)  CountResetPort=on  CountLoadPort=off  CountEnbPort=on  CountDirPort=off  CountDataType=Unsigned  CountWordLen=10  CountFracLen=0  CountSampTime=1e-08
  Initial_Val : Constant  Value=0  OutDataTypeStr=boolean  SampleTime=1e-08
  Logical Operator10 : Logic  AllPortsSameDT=off  OutDataTypeStr=boolean  SampleTime=1e-08
  PipelineDelay1 : Delay  DelayLength=double(1)  InitialCondition=0  SampleTime=1e-08
  Relational Operator : RelationalOperator  Operator===  OutDataTypeStr=boolean  SampleTime=1e-08  RndMeth=Nearest
  Switch : Switch  Criteria=u2 ~= 0  Threshold=double(0)  OutDataTypeStr=boolean  SampleTime=1e-08
  reset_in : Switch  Criteria=u2 ~= 0  Threshold=double(0)  OutDataTypeStr=boolean  SampleTime=1e-08
  reset_out : Switch  Criteria=u2 ~= 0  Threshold=double(0)  OutDataTypeStr=boolean  SampleTime=1e-08
  gate_delay_out : Outport
  wires:
  In1/1 -> Logical Operator10/1, Switch/1, HDL Counter/2, Detect Fall Nonpositive2/1
  DelayCycles/1 -> Relational Operator/1
  Switch/1 -> Logical Operator10/2, reset_in/3
  Relational Operator/1 -> Switch/2
  PipelineDelay1/1 -> reset_out/2, reset_in/2, HDL Counter/1
  Logical Operator10/1 -> gate_delay_out/1
  HDL Counter/1 -> Relational Operator/2
  Detect Fall Nonpositive2/1 -> PipelineDelay1/1
  reset_out/1 -> Switch/3
  Initial_Val/1 -> reset_out/1, reset_in/1
  Delay2_lowered/1 -> reset_out/3
  reset_in/1 -> Delay2_lowered/1

== system gm_interlock_deadtime_vnl/interlock_deadtime/DeadtimeModule_instance6 ==
  In1 : Inport  OutDataTypeStr=boolean  PortDimensions=1  SampleTime=1e-08
  DelayCycles : Inport  Port=2  OutDataTypeStr=fixdt(0, 10, 0)  PortDimensions=1  SampleTime=1e-08
  Delay2_lowered : Delay  DelayLength=double(1)  InitialCondition=0  SampleTime=1e-08
  Detect Fall Nonpositive2 : simulink/Logic and Bit Operations/Detect Fall Nonpositive  vinit=0  OutDataTypeStr=boolean
      settings: SourceProductBaseCode=SL
  HDL Counter : hdlsllib/Sources/HDL Counter  CountType=Free running  CountInit=double(0)  CountStep=double(1)  CountMax=25  CountFromType=Initial value  CountFrom=double(0)  CountResetPort=on  CountLoadPort=off  CountEnbPort=on  CountDirPort=off  CountDataType=Unsigned  CountWordLen=10  CountFracLen=0  CountSampTime=1e-08
  Initial_Val : Constant  Value=0  OutDataTypeStr=boolean  SampleTime=1e-08
  Logical Operator10 : Logic  AllPortsSameDT=off  OutDataTypeStr=boolean  SampleTime=1e-08
  PipelineDelay1 : Delay  DelayLength=double(1)  InitialCondition=0  SampleTime=1e-08
  Relational Operator : RelationalOperator  Operator===  OutDataTypeStr=boolean  SampleTime=1e-08  RndMeth=Nearest
  Switch : Switch  Criteria=u2 ~= 0  Threshold=double(0)  OutDataTypeStr=boolean  SampleTime=1e-08
  reset_in : Switch  Criteria=u2 ~= 0  Threshold=double(0)  OutDataTypeStr=boolean  SampleTime=1e-08
  reset_out : Switch  Criteria=u2 ~= 0  Threshold=double(0)  OutDataTypeStr=boolean  SampleTime=1e-08
  gate_delay_out : Outport
  wires:
  In1/1 -> Logical Operator10/1, Switch/1, HDL Counter/2, Detect Fall Nonpositive2/1
  DelayCycles/1 -> Relational Operator/1
  Switch/1 -> Logical Operator10/2, reset_in/3
  Relational Operator/1 -> Switch/2
  PipelineDelay1/1 -> reset_out/2, reset_in/2, HDL Counter/1
  Logical Operator10/1 -> gate_delay_out/1
  HDL Counter/1 -> Relational Operator/2
  Detect Fall Nonpositive2/1 -> PipelineDelay1/1
  reset_out/1 -> Switch/3
  Initial_Val/1 -> reset_out/1, reset_in/1
  Delay2_lowered/1 -> reset_out/3
  reset_in/1 -> Delay2_lowered/1

== system gm_interlock_deadtime_vnl/interlock_deadtime/EnableOutputModule_instance1 ==
  gate_delay_out : Inport  OutDataTypeStr=boolean  PortDimensions=1  SampleTime=1e-08
  enable : Inport  Port=2  OutDataTypeStr=boolean  PortDimensions=1  SampleTime=1e-08
  AND : Logic  AllPortsSameDT=off  OutDataTypeStr=boolean  SampleTime=1e-08
  gate_enable_out : Outport
  wires:
  AND/1 -> gate_enable_out/1
  enable/1 -> AND/2
  gate_delay_out/1 -> AND/1

== system gm_interlock_deadtime_vnl/interlock_deadtime/EnableOutputModule_instance2 ==
  gate_delay_out : Inport  OutDataTypeStr=boolean  PortDimensions=1  SampleTime=1e-08
  enable : Inport  Port=2  OutDataTypeStr=boolean  PortDimensions=1  SampleTime=1e-08
  AND : Logic  AllPortsSameDT=off  OutDataTypeStr=boolean  SampleTime=1e-08
  gate_enable_out : Outport
  wires:
  gate_delay_out/1 -> AND/1
  enable/1 -> AND/2
  AND/1 -> gate_enable_out/1

== system gm_interlock_deadtime_vnl/interlock_deadtime/EnableOutputModule_instance3 ==
  gate_delay_out : Inport  OutDataTypeStr=boolean  PortDimensions=1  SampleTime=1e-08
  enable : Inport  Port=2  OutDataTypeStr=boolean  PortDimensions=1  SampleTime=1e-08
  AND : Logic  AllPortsSameDT=off  OutDataTypeStr=boolean  SampleTime=1e-08
  gate_enable_out : Outport
  wires:
  gate_delay_out/1 -> AND/1
  enable/1 -> AND/2
  AND/1 -> gate_enable_out/1

== system gm_interlock_deadtime_vnl/interlock_deadtime/EnableOutputModule_instance4 ==
  gate_delay_out : Inport  OutDataTypeStr=boolean  PortDimensions=1  SampleTime=1e-08
  enable : Inport  Port=2  OutDataTypeStr=boolean  PortDimensions=1  SampleTime=1e-08
  AND : Logic  AllPortsSameDT=off  OutDataTypeStr=boolean  SampleTime=1e-08
  gate_enable_out : Outport
  wires:
  gate_delay_out/1 -> AND/1
  enable/1 -> AND/2
  AND/1 -> gate_enable_out/1

== system gm_interlock_deadtime_vnl/interlock_deadtime/EnableOutputModule_instance5 ==
  gate_delay_out : Inport  OutDataTypeStr=boolean  PortDimensions=1  SampleTime=1e-08
  enable : Inport  Port=2  OutDataTypeStr=boolean  PortDimensions=1  SampleTime=1e-08
  AND : Logic  AllPortsSameDT=off  OutDataTypeStr=boolean  SampleTime=1e-08
  gate_enable_out : Outport
  wires:
  gate_delay_out/1 -> AND/1
  enable/1 -> AND/2
  AND/1 -> gate_enable_out/1

== system gm_interlock_deadtime_vnl/interlock_deadtime/EnableOutputModule_instance6 ==
  gate_delay_out : Inport  OutDataTypeStr=boolean  PortDimensions=1  SampleTime=1e-08
  enable : Inport  Port=2  OutDataTypeStr=boolean  PortDimensions=1  SampleTime=1e-08
  AND : Logic  AllPortsSameDT=off  OutDataTypeStr=boolean  SampleTime=1e-08
  gate_enable_out : Outport
  wires:
  gate_delay_out/1 -> AND/1
  enable/1 -> AND/2
  AND/1 -> gate_enable_out/1

== system gm_interlock_deadtime_vnl/interlock_deadtime/InterlockModule_instance1 ==
  In1 : Inport  OutDataTypeStr=boolean  PortDimensions=[2]  SampleTime=1e-08
  In1_0_wire : hdlmdlgenlib/Buffer
      settings: SourceProductBaseCode=SL
  In1_1_wire : hdlmdlgenlib/Buffer
      settings: SourceProductBaseCode=SL
  Logical Operator1 : Logic  AllPortsSameDT=off  OutDataTypeStr=boolean  SampleTime=1e-08
  Logical Operator2 : Logic  AllPortsSameDT=off  OutDataTypeStr=boolean  SampleTime=1e-08
  Logical Operator3 : Logic  Operator=NOT  Inputs=1  AllPortsSameDT=off  OutDataTypeStr=boolean  SampleTime=1e-08
  Logical Operator4 : Logic  Operator=NOT  Inputs=1  AllPortsSameDT=off  OutDataTypeStr=boolean  SampleTime=1e-08
  mux : Mux  Inputs=2
  t : Demux  Outputs=2
  gate_delay_out : Outport
  wires:
  t/2 -> In1_1_wire/1
  t/1 -> In1_0_wire/1
  In1_1_wire/1 -> Logical Operator3/1, Logical Operator1/2
  In1_0_wire/1 -> Logical Operator4/1, Logical Operator2/1
  Logical Operator1/1 -> mux/2
  Logical Operator2/1 -> mux/1
  Logical Operator3/1 -> Logical Operator2/2
  Logical Operator4/1 -> Logical Operator1/1
  mux/1 -> gate_delay_out/1
  In1/1 -> t/1

== system gm_interlock_deadtime_vnl/interlock_deadtime/InterlockModule_instance2 ==
  In1 : Inport  OutDataTypeStr=boolean  PortDimensions=[2]  SampleTime=1e-08
  In1_0_wire : hdlmdlgenlib/Buffer
      settings: SourceProductBaseCode=SL
  In1_1_wire : hdlmdlgenlib/Buffer
      settings: SourceProductBaseCode=SL
  Logical Operator1 : Logic  AllPortsSameDT=off  OutDataTypeStr=boolean  SampleTime=1e-08
  Logical Operator2 : Logic  AllPortsSameDT=off  OutDataTypeStr=boolean  SampleTime=1e-08
  Logical Operator3 : Logic  Operator=NOT  Inputs=1  AllPortsSameDT=off  OutDataTypeStr=boolean  SampleTime=1e-08
  Logical Operator4 : Logic  Operator=NOT  Inputs=1  AllPortsSameDT=off  OutDataTypeStr=boolean  SampleTime=1e-08
  mux : Mux  Inputs=2
  t : Demux  Outputs=2
  gate_delay_out : Outport
  wires:
  In1/1 -> t/1
  mux/1 -> gate_delay_out/1
  Logical Operator4/1 -> Logical Operator1/1
  Logical Operator3/1 -> Logical Operator2/2
  Logical Operator2/1 -> mux/1
  Logical Operator1/1 -> mux/2
  In1_0_wire/1 -> Logical Operator2/1, Logical Operator4/1
  In1_1_wire/1 -> Logical Operator1/2, Logical Operator3/1
  t/1 -> In1_0_wire/1
  t/2 -> In1_1_wire/1

== system gm_interlock_deadtime_vnl/interlock_deadtime/InterlockModule_instance3 ==
  In1 : Inport  OutDataTypeStr=boolean  PortDimensions=[2]  SampleTime=1e-08
  In1_0_wire : hdlmdlgenlib/Buffer
      settings: SourceProductBaseCode=SL
  In1_1_wire : hdlmdlgenlib/Buffer
      settings: SourceProductBaseCode=SL
  Logical Operator1 : Logic  AllPortsSameDT=off  OutDataTypeStr=boolean  SampleTime=1e-08
  Logical Operator2 : Logic  AllPortsSameDT=off  OutDataTypeStr=boolean  SampleTime=1e-08
  Logical Operator3 : Logic  Operator=NOT  Inputs=1  AllPortsSameDT=off  OutDataTypeStr=boolean  SampleTime=1e-08
  Logical Operator4 : Logic  Operator=NOT  Inputs=1  AllPortsSameDT=off  OutDataTypeStr=boolean  SampleTime=1e-08
  mux : Mux  Inputs=2
  t : Demux  Outputs=2
  gate_delay_out : Outport
  wires:
  In1/1 -> t/1
  mux/1 -> gate_delay_out/1
  Logical Operator4/1 -> Logical Operator1/1
  Logical Operator3/1 -> Logical Operator2/2
  Logical Operator2/1 -> mux/1
  Logical Operator1/1 -> mux/2
  In1_0_wire/1 -> Logical Operator2/1, Logical Operator4/1
  In1_1_wire/1 -> Logical Operator1/2, Logical Operator3/1
  t/1 -> In1_0_wire/1
  t/2 -> In1_1_wire/1
